simulink model "MODAL2"  (R2013a)
settings: Solver=ode45  StartTime=0.0  StopTime=10.0  RelTol=1e-3
values from neighbouring files (symbols this model uses):
  f = 7.26e-3    (= 0.00726)    [parametres.m]
  g1 = K/Kh + l2 + R*f/(K*Kh) + l1*f/K    (= 0.000102484459459)    [parametres.m]
  g2 = R/(Kh*K) + l1/K    (= 0.0019285625889)    [parametres.m]
  J = 0.038    [parametres.m]
  K = 0.74    [parametres.m]
  K1 = Kh*l1    (= -0.265728636842)    [parametres.m]
  K2 = -Kh*l2    (= 0.739115169049)    [parametres.m]
  Kh = 10    [parametres.m]
  L = 8.87e-3    (= 0.00887)    [parametres.m]
  l1 = (L*(2*Csi*w0 - f/J)-R)/Kh    (= -0.0265728636842)    [parametres.m]
  l2 = (w0^2*L*J - f*(R+Kh*l1) - K^2)/(Kh*K)    (= -0.0739115169049)    [parametres.m]
  R = 0.28    [parametres.m]
settings Model: Creator=ciottopinton_gus  LastModifiedBy=ciottopinton_gus

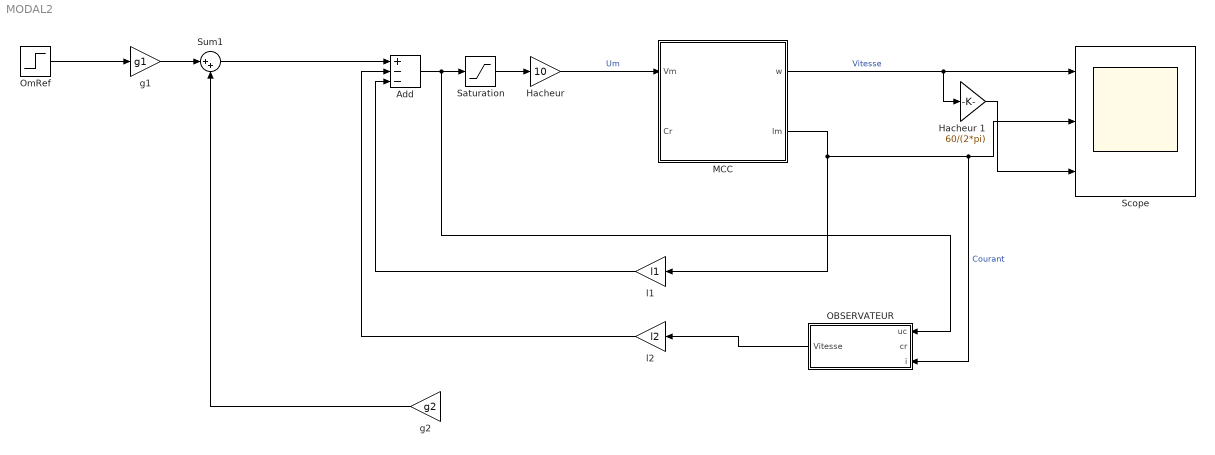
== system MODAL2 ==
  Add : Sum  Inputs=+--
  "Hacheur " : Gain  Gain=10
  Hacheur 1 : Gain  Gain=60/(2*pi)
  MCC : Subsystem
  OBSERVATEUR : Subsystem
  OmRef : Step  Time=0  After=800*2*pi/60  SampleTime=0
  Saturation : Saturate  UpperLimit=9  LowerLimit=-9
  Scope : Scope  NumInputPorts=3
      settings: YMin=-5~-5~-5  YMax=5~5~5
  Sum1 : Sum  Inputs=|++
  g1 : Gain  Gain=g1
  "g2 " : Gain  Gain=g2
  l1 : Gain  Gain=l1
  l2 : Gain  Gain=l2
  wires:
  "Hacheur "/1 -> MCC/1("Vm ")  "Um"
  Saturation/1 -> "Hacheur "/1
  Add/1 -> OBSERVATEUR/1(uc), Saturation/1
  ? -> OBSERVATEUR/2(cr), "g2 "/1, MCC/2("Cr ")
  l1/1 -> Add/3
  l2/1 -> Add/2
  MCC/2(Im) -> OBSERVATEUR/3(i), Scope/2, l1/1  "Courant"
  MCC/1(w) -> Scope/1, Hacheur 1/1  "Vitesse"
  Hacheur 1/1 -> Scope/3
  OmRef/1 -> g1/1
  g1/1 -> Sum1/1
  "g2 "/1 -> Sum1/2
  Sum1/1 -> Add/1
  OBSERVATEUR/1(Vitesse) -> l2/1

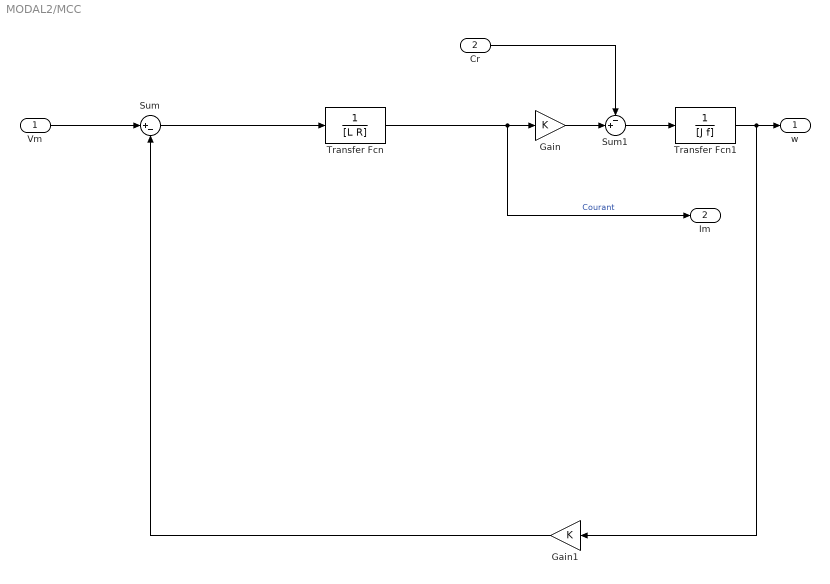
== system MODAL2/MCC ==
  "Vm " : Inport
  "Cr " : Inport  Port=2
  Gain : Gain  Gain=K
  Gain1 : Gain  Gain=K
  Sum : Sum  Inputs=|+-
  Sum1 : Sum  Inputs=-+|
  Transfer Fcn : TransferFcn  Denominator=[L R]
  Transfer Fcn1 : TransferFcn  Denominator=[J f]
  w : Outport
  Im : Outport  Port=2
  wires:
  "Vm "/1 -> Sum/1
  Gain/1 -> Sum1/2
  "Cr "/1 -> Sum1/1
  Sum1/1 -> Transfer Fcn1/1
  Transfer Fcn1/1 -> Gain1/1, w/1
  Gain1/1 -> Sum/2
  Transfer Fcn/1 -> Im/1, Gain/1  "Courant"
  Sum/1 -> Transfer Fcn/1

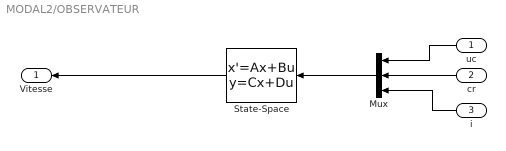
== system MODAL2/OBSERVATEUR ==
  uc : Inport
  cr : Inport  Port=2
  i : Inport  Port=3
  Mux : Mux  Inputs=3
  State-Space : StateSpace  A="[ [-(R + K1)/L  -K/L] ; [ (K - K2)/J -f/J ] ]"  B="[ [Kh/L 0 K1/L] ; [ 0 -1/J  K2/J ] ]"  C=[ 0 1 ]  D=[ 0 0 0 ]
  Vitesse : Outport
  wires:
  Mux/1 -> State-Space/1
  i/1 -> Mux/3
  cr/1 -> Mux/2
  uc/1 -> Mux/1
  State-Space/1 -> Vitesse/1
